simulink model "CH7_2"  (Simulink 7.5)
settings: Solver=ode45  StartTime=0.0  StopTime=20  RelTol=1e-3
libraries: dsparch4 x1
settings Model: Creator=xnote  LastModifiedBy=xnote

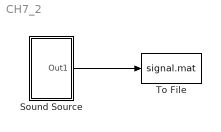
== system CH7_2 ==
  Sound Source : Subsystem
  To File : ToFile  Filename=signal.mat  SampleTime=1/8192
  wires:
  Sound Source/1(Out1) -> To File/1

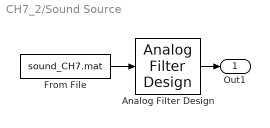
== system CH7_2/Sound Source ==
  Analog Filter Design : dsparch4/Analog Filter Design  method=Butterworth  filttype=Lowpass  N=8  Wlo=2*pi*4e3  Whi=80  Rp=2  Rs=40
  From File : FromFile  FileName=sound_CH7.mat  SampleTime=0
  Out1 : Outport
  wires:
  From File/1 -> Analog Filter Design/1
  Analog Filter Design/1 -> Out1/1
